simulink model "viena_model"  (R2018a)
settings: Solver=ode45  StartTime=0.0  StopTime=t_max  RelTol=1e-5
values from neighbouring files (symbols this model uses):
  A = 1.508*1.420    (= 2.14136)    [run.m]
  Cd = 0.33    [run.m]
  EQSolutions = @(v,f,r) motor.EQSolutions(v,f,r)    [run.m]
  fr = 0.01    [run.m]
  g = 9.81    [run.m]
  lf = 3.23/2    (= 1.615)    [run.m]
  lr = 3.23/2    (= 1.615)    [run.m]
  m = 700+2*70    (= 840)    [run.m]
  pp = 2    [run.m]
  rho = Press/(R*Tar)    (= 1.29295768156)    [run.m]
  rw = 0.1651    [run.m]
  t_sample = 1    [run.m]
  V_F = 1    [run.m]
libraries: simulink x3
settings Model: Creator=João Fernandes  LastModifiedBy=Francisco

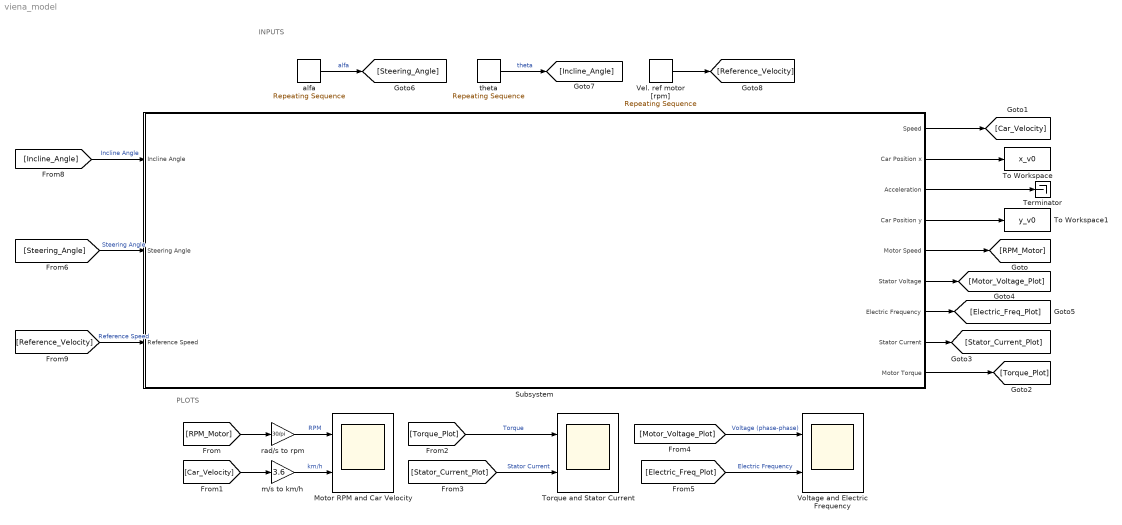
== system viena_model ==
  note: INPUTS
  note: PLOTS
  Motor RPM and Car Velocity : Scope  NumInputPorts=2
  Subsystem : Subsystem
      mask Display: image('vienalogo.jpg');
  Terminator : Terminator
  To Workspace : ToWorkspace  VariableName=x_v0  SaveFormat=Timeseries  SampleTime=t_sample
  To Workspace1 : ToWorkspace  VariableName=y_v0  SaveFormat=Timeseries  SampleTime=t_sample
  Torque and Stator Current : Scope  NumInputPorts=2
  Vel. ref motor [rpm] : simulink/Sources/Repeating Sequence  rep_seq_t=v_t  rep_seq_y=v_v
  Voltage and Electric Frequency : Scope  NumInputPorts=2
  alfa : simulink/Sources/Repeating Sequence  rep_seq_t=alfa_t  rep_seq_y=alfa_v
  m/s to km/h : Gain  Gain=3.6
  rad/s to rpm : Gain  Gain=30/pi
  theta : simulink/Sources/Repeating Sequence  rep_seq_t=theta_t  rep_seq_y=theta_v
  wires:
  alfa/1 -> [Steering_Angle]  "alfa"
  [RPM_Motor] -> rad/s to rpm/1
  [Car_Velocity] -> m/s to km/h/1
  m/s to km/h/1 -> Motor RPM and Car Velocity/2  "km/h"
  rad/s to rpm/1 -> Motor RPM and Car Velocity/1  "RPM"
  [Torque_Plot] -> Torque and Stator Current/1  "Torque"
  [Stator_Current_Plot] -> Torque and Stator Current/2  "Stator Current"
  [Motor_Voltage_Plot] -> Voltage and Electric Frequency/1  "Voltage (phase-phase)"
  [Electric_Freq_Plot] -> Voltage and Electric Frequency/2  "Electric Frequency"
  theta/1 -> [Incline_Angle]  "theta"
  Vel. ref motor [rpm]/1 -> [Reference_Velocity]
  [Incline_Angle] -> Subsystem/1(Incline Angle)  "Incline Angle"
  [Steering_Angle] -> Subsystem/2(Steering Angle)  "Steering Angle"
  [Reference_Velocity] -> Subsystem/3(Reference Speed)  "Reference Speed"
  Subsystem/1(Speed) -> [Car_Velocity]
  Subsystem/2(Car Position x) -> To Workspace/1
  Subsystem/3(Acceleration) -> Terminator/1
  Subsystem/4(Car Position y) -> To Workspace1/1
  Subsystem/5(Motor Speed) -> [RPM_Motor]
  Subsystem/6(Stator Voltage) -> [Motor_Voltage_Plot]
  Subsystem/7(Electric Frequency) -> [Electric_Freq_Plot]
  Subsystem/8(Stator Current) -> [Stator_Current_Plot]
  Subsystem/9(Motor Torque) -> [Torque_Plot]

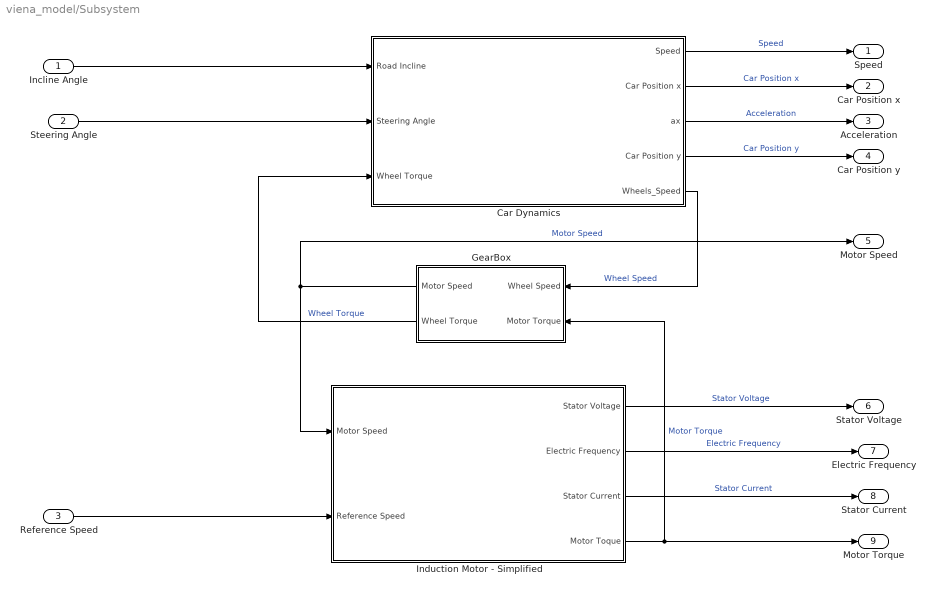
== system viena_model/Subsystem ==
  Incline Angle : Inport
  Steering Angle : Inport  Port=2
  Reference Speed : Inport  Port=3
  Car Dynamics : Subsystem
      mask Display: image('porche.jpg');
  GearBox : Subsystem
  Induction Motor - Simplified : Subsystem
      mask Display: image('Induction_Motor.jpg');
  Speed : Outport
  Car Position x : Outport  Port=2
  Acceleration : Outport  Port=3
  Car Position y : Outport  Port=4
  Motor Speed : Outport  Port=5
  Stator Voltage : Outport  Port=6
  Electric Frequency : Outport  Port=7
  Stator Current : Outport  Port=8
  Motor Torque : Outport  Port=9
  wires:
  GearBox/1("Motor Speed ") -> Motor Speed/1, Induction Motor - Simplified/1(Motor Speed)  "Motor Speed"
  GearBox/2(Wheel Torque) -> Car Dynamics/3(Wheel Torque)  "Wheel Torque"
  Incline Angle/1 -> Car Dynamics/1(Road Incline)
  Induction Motor - Simplified/1(Stator Voltage) -> Stator Voltage/1  "Stator Voltage"
  Car Dynamics/1(Speed) -> Speed/1  "Speed"
  Car Dynamics/5(Wheels_Speed) -> GearBox/1(Wheel Speed)  "Wheel Speed"
  Induction Motor - Simplified/2(Electric Frequency) -> Electric Frequency/1  "Electric Frequency"
  Induction Motor - Simplified/4(Motor Toque) -> Motor Torque/1, GearBox/2(Motor Torque)  "Motor Torque"
  Car Dynamics/2(Car Position x) -> Car Position x/1  "Car Position x"
  Steering Angle/1 -> Car Dynamics/2(Steering Angle)
  Car Dynamics/4(Car Position y) -> Car Position y/1  "Car Position y"
  Induction Motor - Simplified/3(Stator Current) -> Stator Current/1  "Stator Current"
  Reference Speed/1 -> Induction Motor - Simplified/2(Reference Speed)
  Car Dynamics/3(ax) -> Acceleration/1  "Acceleration"

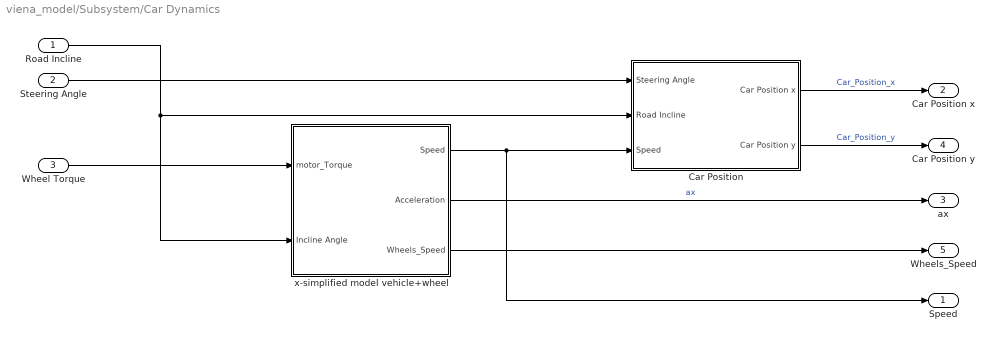
== system viena_model/Subsystem/Car Dynamics ==
  Road Incline : Inport
  Steering Angle : Inport  Port=2
  Wheel Torque : Inport  Port=3
  Car Position : Subsystem
  x-simplified model vehicle+wheel : Subsystem
  Speed : Outport
  Car Position x : Outport  Port=2
  ax : Outport  Port=3
  Car Position y : Outport  Port=4
  Wheels_Speed : Outport  Port=5
  wires:
  Wheel Torque/1 -> x-simplified model vehicle+wheel/1(motor_Torque)
  x-simplified model vehicle+wheel/1(Speed) -> Speed/1, Car Position/3(Speed)
  x-simplified model vehicle+wheel/2(Acceleration) -> ax/1  "ax"
  Steering Angle/1 -> Car Position/1(Steering Angle)
  Car Position/2(Car Position y) -> Car Position y/1  "Car_Position_y"
  Road Incline/1 -> x-simplified model vehicle+wheel/2(Incline Angle), Car Position/2(Road Incline)
  x-simplified model vehicle+wheel/3(Wheels_Speed) -> Wheels_Speed/1
  Car Position/1(Car Position x) -> Car Position x/1  "Car_Position_x"

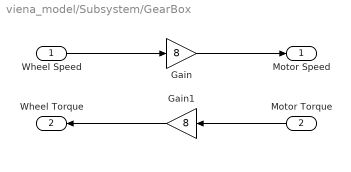
== system viena_model/Subsystem/GearBox ==
  Wheel Speed : Inport
  Motor Torque : Inport  Port=2
  Gain : Gain  Gain=8
  Gain1 : Gain  Gain=8
  "Motor Speed " : Outport
  Wheel Torque : Outport  Port=2
  wires:
  Wheel Speed/1 -> Gain/1
  Gain/1 -> "Motor Speed "/1
  Motor Torque/1 -> Gain1/1
  Gain1/1 -> Wheel Torque/1

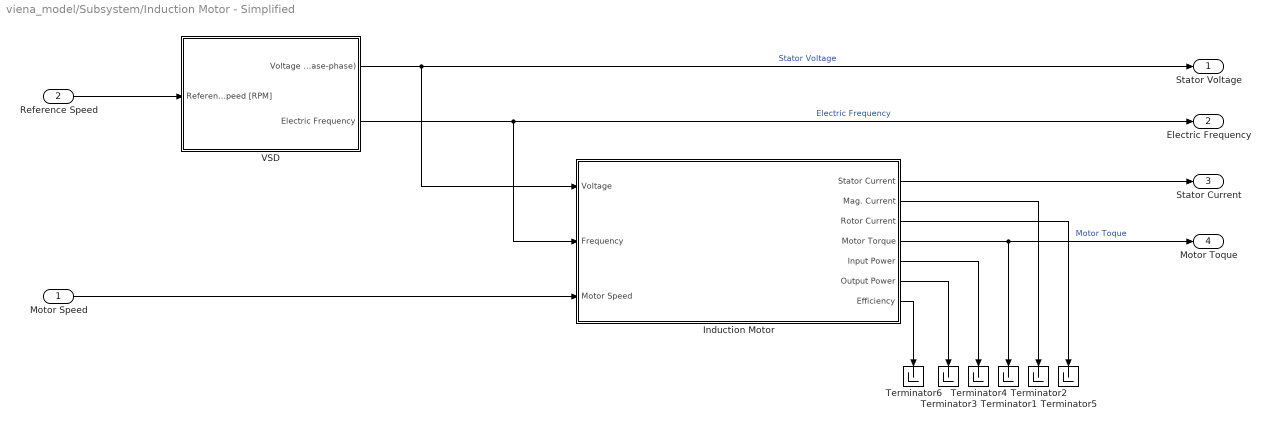
== system viena_model/Subsystem/Induction Motor - Simplified ==
  Motor Speed : Inport
  Reference Speed : Inport  Port=2
  Induction Motor : Subsystem
  Terminator{1..6} (6 alike) : Terminator
  VSD : Subsystem
  Stator Voltage : Outport
  Electric Frequency : Outport  Port=2
  Stator Current : Outport  Port=3
  Motor Toque : Outport  Port=4
  wires:
  Induction Motor/2(Mag. Current) -> Terminator2/1
  VSD/2(Electric Frequency) -> Electric Frequency/1, Induction Motor/2(Frequency)  "Electric Frequency"
  VSD/1(Voltage (phase-phase)) -> Stator Voltage/1, Induction Motor/1(Voltage)  "Stator Voltage"
  Induction Motor/6(Output Power) -> Terminator3/1
  Motor Speed/1 -> Induction Motor/3(Motor Speed)
  Induction Motor/5(Input Power) -> Terminator4/1
  Reference Speed/1 -> VSD/1(Reference_Speed [RPM])
  Induction Motor/3(Rotor Current) -> Terminator5/1
  Induction Motor/7(Efficiency) -> Terminator6/1
  Induction Motor/1(Stator Current) -> Stator Current/1
  Induction Motor/4(Motor Torque) -> Terminator1/1, Motor Toque/1  "Motor Toque"

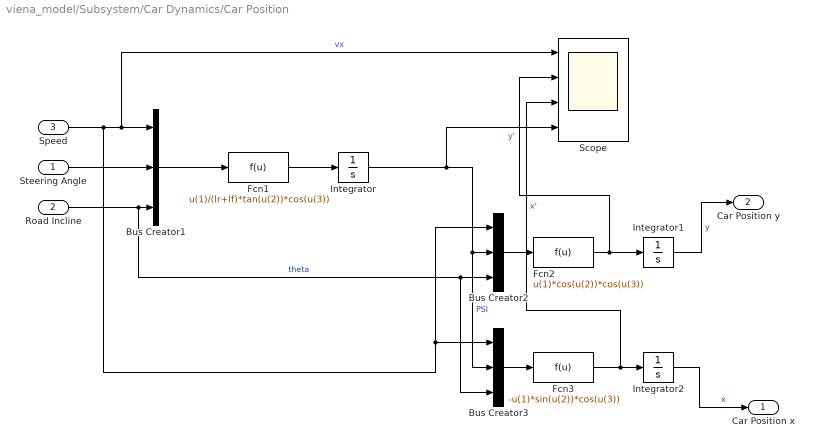
== system viena_model/Subsystem/Car Dynamics/Car Position ==
  Steering Angle : Inport
  Road Incline : Inport  Port=2
  Speed : Inport  Port=3
  Bus Creator1 : BusCreator  Inputs=3
  Bus Creator2 : BusCreator  Inputs=3
  Bus Creator3 : BusCreator  Inputs=3
  Fcn1 : Fcn  Expr=u(1)/(lr+lf)*tan(u(2))*cos(u(3))
  Fcn2 : Fcn  Expr=u(1)*cos(u(2))*cos(u(3))
  Fcn3 : Fcn  Expr=-u(1)*sin(u(2))*cos(u(3))
  Integrator : Integrator
  Integrator1 : Integrator
  Integrator2 : Integrator
  Scope : Scope  NumInputPorts=4
  Car Position x : Outport
  Car Position y : Outport  Port=2
  wires:
  Integrator1/1 -> Car Position y/1  "y"
  Integrator2/1 -> Car Position x/1  "x"
  Road Incline/1 -> Bus Creator3/3, Bus Creator2/3, Bus Creator1/3  "theta"
  Bus Creator1/1 -> Fcn1/1
  Fcn1/1 -> Integrator/1
  Bus Creator2/1 -> Fcn2/1
  Speed/1 -> Bus Creator2/1, Bus Creator3/1, Scope/1, Bus Creator1/1  "vx"
  Fcn2/1 -> Scope/2, Integrator1/1  "y'"
  Fcn3/1 -> Scope/3, Integrator2/1  "x'"
  Integrator/1 -> Scope/4, Bus Creator3/2, Bus Creator2/2  "PSI"
  Bus Creator3/1 -> Fcn3/1
  Steering Angle/1 -> Bus Creator1/2

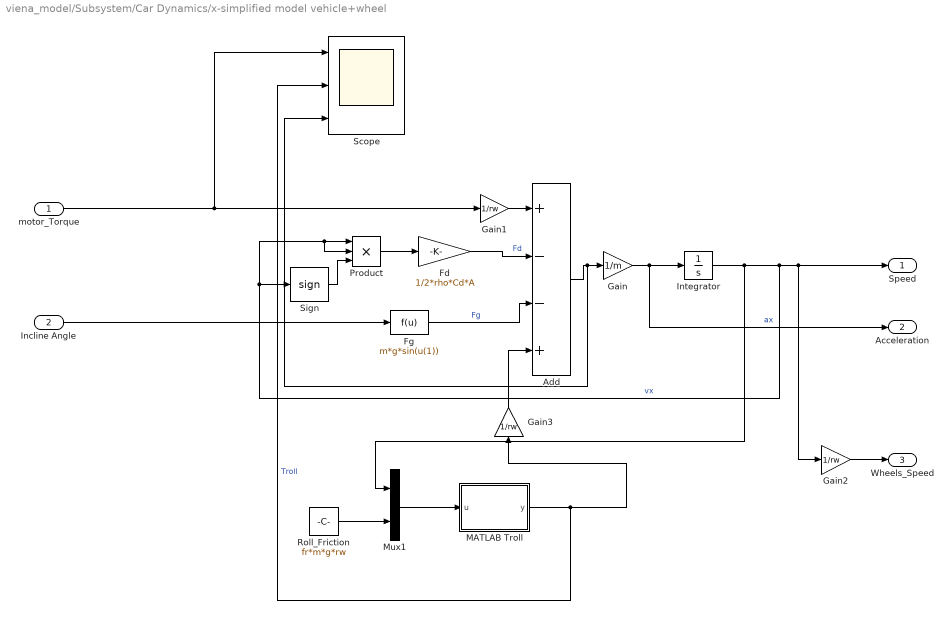
== system viena_model/Subsystem/Car Dynamics/x-simplified model vehicle+wheel ==
  motor_Torque : Inport
  Incline Angle : Inport  Port=2
  Add : Sum  Inputs=+--+
  Fd : Gain  Gain=1/2*rho*Cd*A
  Fg : Fcn  Expr=m*g*sin(u(1))
  Gain : Gain  Gain=1/m
  Gain1 : Gain  Gain=1/rw
  Gain2 : Gain  Gain=1/rw
  Gain3 : Gain  Gain=1/rw
  Integrator : Integrator
  MATLAB Troll : MATLAB Function  TreatAsAtomicUnit=on
  Mux1 : Mux  Inputs=2
  Product : Product  Inputs=3
  "Roll_Friction " : Constant  Value=fr*m*g*rw
  Scope : Scope  NumInputPorts=3
  Sign : Signum
  Speed : Outport
  Acceleration : Outport  Port=2
  Wheels_Speed : Outport  Port=3
  wires:
  Product/1 -> Fd/1
  Incline Angle/1 -> Fg/1
  Fg/1 -> Add/3  "Fg"
  Add/1 -> Scope/3, Gain/1
  Gain/1 -> Integrator/1, Acceleration/1  "ax"
  Fd/1 -> Add/2  "Fd"
  Integrator/1 -> Mux1/1, Gain2/1, Speed/1, Sign/1, Product/2, Product/1  "vx"
  Sign/1 -> Product/3
  Gain1/1 -> Add/1
  Gain2/1 -> Wheels_Speed/1
  motor_Torque/1 -> Scope/1, Gain1/1
  "Roll_Friction "/1 -> Mux1/2
  Mux1/1 -> MATLAB Troll/1(u)
  MATLAB Troll/1(y) -> Scope/2, Gain3/1  "Troll"
  Gain3/1 -> Add/4

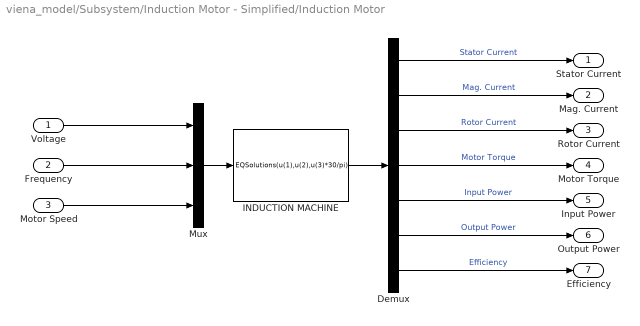
== system viena_model/Subsystem/Induction Motor - Simplified/Induction Motor ==
  Voltage : Inport
  Frequency : Inport  Port=2
  Motor Speed : Inport  Port=3
  Demux : Demux  Outputs=7
  INDUCTION MACHINE : MATLABFcn  MATLABFcn=EQSolutions(u(1),u(2),u(3)*30/pi)  OutputDimensions=7  OutputSignalType=real  Output1D=off  mask(Induction Motor){}
  Mux : Mux  Inputs=3
  Stator Current : Outport
  Mag. Current : Outport  Port=2
  Rotor Current : Outport  Port=3
  Motor Torque : Outport  Port=4
  Input Power : Outport  Port=5
  Output Power : Outport  Port=6
  Efficiency : Outport  Port=7
  wires:
  Frequency/1 -> Mux/2
  Demux/3 -> Rotor Current/1  "Rotor Current"
  Demux/6 -> Output Power/1  "Output Power"
  Demux/4 -> Motor Torque/1  "Motor Torque"
  Demux/7 -> Efficiency/1  "Efficiency"
  INDUCTION MACHINE/1 -> Demux/1
  Mux/1 -> INDUCTION MACHINE/1
  Demux/5 -> Input Power/1  "Input Power"
  Demux/2 -> Mag. Current/1  "Mag. Current"
  Motor Speed/1 -> Mux/3
  Demux/1 -> Stator Current/1  "Stator Current"
  Voltage/1 -> Mux/1

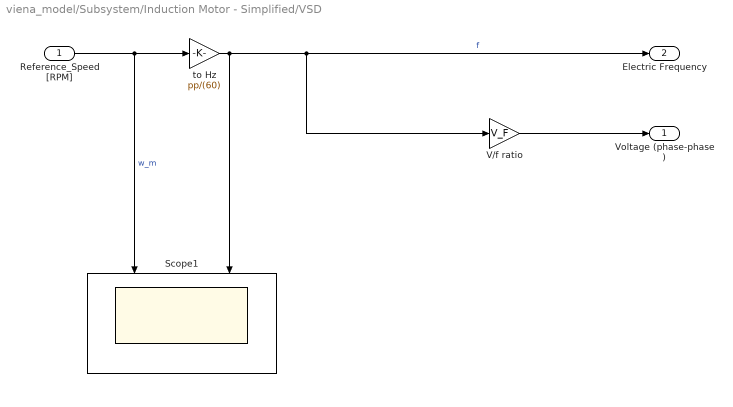
== system viena_model/Subsystem/Induction Motor - Simplified/VSD ==
  Reference_Speed [RPM] : Inport
  Scope1 : Scope  NumInputPorts=2
  V/f ratio : Gain  Gain=V_F
  to Hz : Gain  Gain=pp/(60)
  Voltage (phase-phase) : Outport
  Electric Frequency : Outport  Port=2
  wires:
  Reference_Speed [RPM]/1 -> to Hz/1, Scope1/1  "w_m"
  to Hz/1 -> Electric Frequency/1, V/f ratio/1, Scope1/2  "f"
  V/f ratio/1 -> Voltage (phase-phase)/1

== matlab function viena_model/Subsystem/Car Dynamics/x-simplified model vehicle+wheel/MATLAB Troll ==
  data: u input; y output
function y = fTout(u)
y=0;
vx=u(1);
Troll=u(2);

if vx>0.01
   y=-Troll; % se o carro estiver a andar para a frente, este atrito trava o movimento
elseif vx<-0.01
    y=Troll; % se o carro estiver a andar para trás, este atrito trava o movimento
else
    y=0;
end
